simulink model "ComputeGammaPower"  (R2016b)
settings: Solver=FixedStepDiscrete  StartTime=0.0  StopTime=inf  FixedStep=sCoreParams.core.stepPeriod  RelTol=1e-3
undefined symbols (not defined in the file): dfilt, sCoreParams, sCoreParams_features_computePower
libraries: dspstat3 x4, dsparch4 x2
settings Model: Creator=anish  LastModifiedBy=rzelmann
settings SolverCC: EnableConcurrentExecution=on
settings DataIOCC: LimitDataPoints=on  SaveFormat=Array  SignalLoggingSaveFormat=ModelDataLogs
settings OptimizationCC: BlockReduction=off  BooleanDataType=off  DefaultParameterBehavior=Inlined  OptimizeBlockIOStorage=off  BufferReuse=off  GlobalBufferReuse=off  ExpressionFolding=off  LocalBlockOutputs=off  LifeSpan=inf
settings DebuggingCC: SaveWithParameterizedLinksMsg=none  UnderspecifiedInitializationDetection=Classic  MergeDetectMultiDrivingBlocksExec=none  SignalResolutionControl=TryResolveAllWithWarning  MultiTaskDSMMsg=warning  MultiTaskCondExecSysMsg=none  StateNameClashWarn=warning  SFUnexpectedBacktrackingDiag=warning  SFNoUnconditionalDefaultTransitionDiag=warning  SFExecutionAtInitializationDiag=none
settings HardwareCC: ProdBitPerPointer=32  ProdBitPerSizeT=32  ProdBitPerPtrDiffT=32  ProdLargestAtomicFloat=None  ProdWordSize=32  ProdLongLongMode=on  ProdHWDeviceType=Generic->32-bit x86 compatible  TargetBitPerPointer=64  TargetBitPerSizeT=64  TargetBitPerPtrDiffT=64  TargetLongLongMode=on  TargetIntDivRoundTo=Zero  TargetEndianess=LittleEndian  TargetWordSize=64  TargetHWDeviceType=MATLAB Host
settings ModelReferenceCC: UpdateModelReferenceTargets=Force  PropagateSignalLabelsOutOfModel=off
settings RTWCC: SystemTargetFile=slrt.tlc  TemplateMakefile=slrt_default_tmf  Description=Simulink Real-Time  RTWCompilerOptimization=on
settings ConfigComp: CovMetricSettings=dw  CovHtmlReporting=on  CovSaveCumulativeToWorkspaceVar=on  CovSaveSingleToWorkspaceVar=on  CovExternalEMLEnable=off

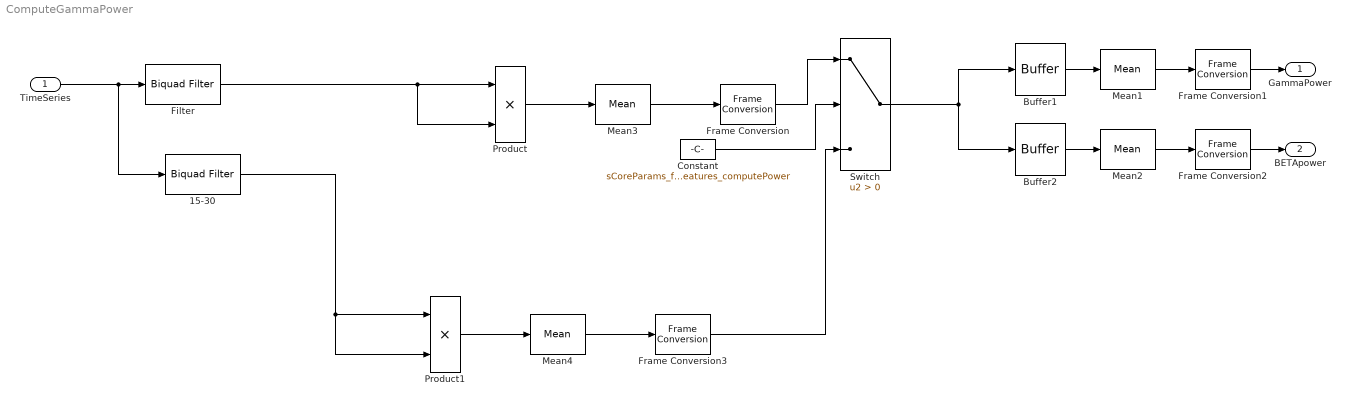
== system ComputeGammaPower ==
  TimeSeries : Inport  PortDimensions=[sCoreParams.core.samplesPerStep sCoreParams.core.maxChannelsPerNSP]  Interpolate=off
  15-30 : dsparch4/Biquad Filter  Tag=BlockMethodSubSystem  IIRFiltStruct=Direct form II  CoeffSource=Specify via dialog  BiQuadCoeffs=[1 0 -1 1 -1.9496142925968893 0.95395255590776118]  a0Flag=Warning  IC=0  ICnum=0  ICden=0  InputProcessing=Columns as channels (frame based)  denAccumFracLength=30  denProdOutputFracLength=30  secondMemoryFracLength=15  roundingMode=Floor  overflowMode=off  ScaleValues=[0.023023722046119379;1]  optimizeScaleValues=off  ScaleValueMode=Specify via input port (g)  scaleValueFracLength=14  FilterSource=Specify via dialog  FilterObject=dfilt.df2tsos([1 0.3 0.4],[1 0.1 0.2])
  Buffer1 : Buffer  N=.05/sCoreParams.core.stepPeriod  V=.05/sCoreParams.core.stepPeriod-1  TreatMby1Signals=One channel
  Buffer2 : Buffer  N=.1/sCoreParams.core.stepPeriod  V=.1/sCoreParams.core.stepPeriod-1  TreatMby1Signals=One channel
  Constant : Constant  Value=sCoreParams_features_computePower
  Filter : dsparch4/Biquad Filter  Tag=BlockMethodSubSystem  IIRFiltStruct=Direct form II  CoeffSource=Specify via dialog  BiQuadCoeffs=[1 0 -1 1 -0.87561361197430121 0.12792556134289804]  a0Flag=Warning  IC=0  ICnum=0  ICden=0  InputProcessing=Columns as channels (frame based)  denAccumFracLength=30  denProdOutputFracLength=30  secondMemoryFracLength=15  roundingMode=Floor  overflowMode=off  ScaleValues=[0.436037219328551;1]  optimizeScaleValues=off  ScaleValueMode=Specify via input port (g)  scaleValueFracLength=14  FilterSource=Specify via dialog  FilterObject=dfilt.df2tsos([1 0.3 0.4],[1 0.1 0.2])
  Frame Conversion{,1..3} (4 alike) : FrameConversion  InheritSamplingMode=off  OutFrame=Sample-based
  Mean{1..4} (4 alike) : dspstat3/Mean  run=off  reset_popup=None  InputProcessing=Columns as channels (frame based)  directionMode=Each column  dimension=1  roiEnable=off  roiType=Rectangles  roiPortion=Entire ROI  roiOutput=Individual statistics for each ROI  roiFlag=off  outputDataTypeStr=Inherit: Same as accumulator  outputLastDataTypeStr=Inherit: Same as accumulator  outputMin=[]  outputMax=[]  roundingMode=Floor  overflowMode=off
  Product : Product
  Product1 : Product
  Switch : Switch  Criteria=u2 > Threshold
  GammaPower : Outport
  BETApower : Outport  Port=2
  wires:
  Filter/1 -> Product/1, Product/2
  Product/1 -> Mean3/1
  Mean3/1 -> Frame Conversion/1
  TimeSeries/1 -> Filter/1, 15-30/1
  Switch/1 -> Buffer2/1, Buffer1/1
  Frame Conversion/1 -> Switch/1
  Constant/1 -> Switch/2
  Buffer1/1 -> Mean1/1
  Mean1/1 -> Frame Conversion1/1
  Frame Conversion1/1 -> GammaPower/1
  Frame Conversion2/1 -> BETApower/1
  Mean2/1 -> Frame Conversion2/1
  Buffer2/1 -> Mean2/1
  Mean4/1 -> Frame Conversion3/1
  Frame Conversion3/1 -> Switch/3
  Product1/1 -> Mean4/1
  15-30/1 -> Product1/2, Product1/1
